simulink model "M10B39_es_V3"  (R2025a)
settings: Solver=ode23tb  StartTime=0.0  StopTime=100  FixedStep=0.001  MaxStep=0.01  RelTol=1e-3  EnableMultiTasking=on
InitFcn:
  | initAll_V3
values from neighbouring files (symbols this model uses):
  acom = 100    [initAll_V1.m]    (also in initAll_V2.m; initAll_V3.m; parameterinit.mat)
  AVm0 = [4.26082678503 4.656135219]    [parameterinit.mat]
  bcom = 50    [initAll_V1.m]    (also in initAll_V2.m; initAll_V3.m; parameterinit.mat)
  commun = 0*commun    [initAll_V1.m]    (also in initAll_V2.m; initAll_V3.m; parameterinit.mat = [0  0  0; 0  0  0; 0  0  0; 0  0  0])
  DataDelay = 0.0*DataDelay    [initAll_V1.m]    (also in initAll_V2.m; initAll_V3.m; parameterinit.mat = [0  0  0; 0  0  0; 0  0  0; 0  0  0])
  ESinit =     [parameterinit.mat]
  fB = 50    [initAll.m]    (also in initAll_V1.m; initAll_V2.m; initAll_V3.m; parameterinit.mat)
  Geninit = Generator_init(opdata,SynMach_in_gidx)    [initAll.m]    (also in initAll_V1.m; initAll_V2.m; initAll_V3.m = Generator_init(opdata_all,SynMach_in_gidx1); parameterinit.mat = )
  lam = 100    [initAll_V1.m]    (also in initAll_V2.m; initAll_V3.m; parameterinit.mat)
  SgridB = 100    [initAll.m]    (also in initAll_V1.m; initAll_V2.m; initAll_V3.m; parameterinit.mat)
  wB = 2*pi*fB    (= 314.159265359)    [initAll.m]    (also in initAll_V1.m; initAll_V2.m; initAll_V3.m; parameterinit.mat)
  Windinit =     [parameterinit.mat]
  YY_load = [3.65450097002 -2.05705688056 0 0 0 0 0 0 0 0 0 0 ... (1521 elements, 39x39)]    [parameterinit.mat]    (also in powerflowcaculate.m = full(YY))
undefined symbols (not defined in the file or in its folder): c1, c2, c3, c4, c5, c6, cp_nom, lambda_nom, P_wind_base, Pelec_base, Pnom
libraries: spsBistableLib x12, simulink_extras x3, slpidlib x2, simulink x1
(part 1 of 7)
settings Model: Creator=m  LastModifiedBy=86182
settings SolverCC: AlgebraicLoopSolver=TrustRegion
settings DataIOCC: LimitDataPoints=on  SaveFormat=Array  SignalLoggingSaveFormat=ModelDataLogs  ReturnWorkspaceOutputs=off  SignalLoggingName=sigsOut
settings OptimizationCC: ExpressionDepthLimit=2147483647.0  LifeSpan=inf
settings DebuggingCC: SaveWithParameterizedLinksMsg=none  UnderspecifiedInitializationDetection=Classic  MergeDetectMultiDrivingBlocksExec=none  SignalResolutionControl=TryResolveAllWithWarning  MultiTaskDSMMsg=warning  MultiTaskCondExecSysMsg=none  FcnCallInpInsideContextMsg=warning  UnconnectedInputMsg=warning  UnconnectedOutputMsg=warning  UnconnectedLineMsg=warning  StateNameClashWarn=warning  SFUnexpectedBacktrackingDiag=warning  SFNoUnconditionalDefaultTransitionDiag=warning  SFExecutionAtInitializationDiag=none  ArithmeticOperatorsInVariantConditions=warning
settings HardwareCC: ProdBitPerPointer=32.0  ProdBitPerSizeT=32.0  ProdBitPerPtrDiffT=32.0  ProdLargestAtomicFloat=None  ProdIntDivRoundTo=Undefined  ProdEndianess=Unspecified  ProdWordSize=32.0  ProdHWDeviceType=32-bit Generic  TargetUnknown=on
settings ModelReferenceCC: EnableRefExpFcnMdlSchedulingChecks=on  PropagateSignalLabelsOutOfModel=off
settings SFSimCC: SimUseLocalCustomCode=off  CustomCodeUndefinedFunction=UseInterfaceOnly
settings RTWCC: RTWUseLocalCustomCode=off  GPUComputeCapability=3.5
settings CodeAppCC: StateflowObjectComments=on
settings GRTTargetCC: TargetLangStandard=C89/C90 (ANSI)  CombineOutputUpdateFcns=off  GRTInterface=on
settings ConfigComp: CovMetricSettings=dw  CovSaveCumulativeToWorkspaceVar=on  CovSaveSingleToWorkspaceVar=on  CovExternalEMLEnable=off  CovSFcnEnable=off

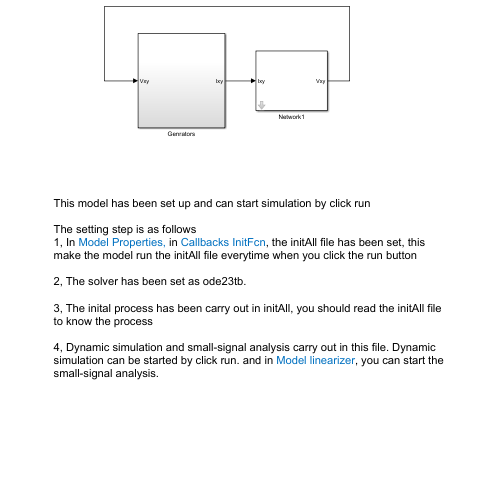
[thumbnail: Simulink's stored preview of the top-level diagram]
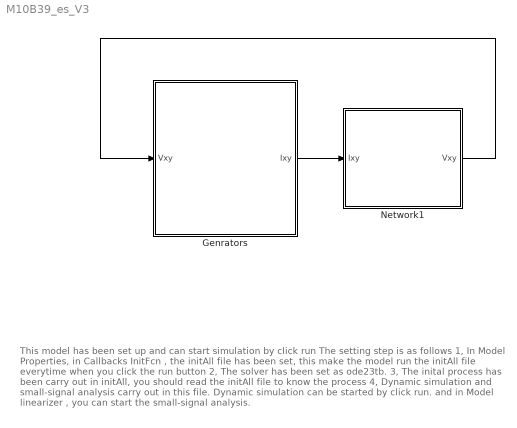
== system M10B39_es_V3 ==
  note: This model has been set up and can start simulation by click run
      |
      | The setting step is as follows
      | 1, In Model Properties, in Callbacks InitFcn , the initAll file has been set, this make the model run the initAll file everytime when you click the run button
      |
      | 2, The solver has been set as ode23tb.
      |
      | 3, The inital process has been carry out in initAll, you should read the initAll file to know the process
      |
      | 4, Dynamic simulation and small-signal analysis carry out in this file. Dynamic simulation can be started by click run. and in Model linearizer , you can start the small-signal analysis.
  Genrators : Subsystem
  Network1 : Subsystem  mask{YY_load=YY_load, ng=12}
  wires:
  Genrators/1(Ixy) -> Network1/1(Ixy)
  Network1/1(Vxy) -> Genrators/1(Vxy)

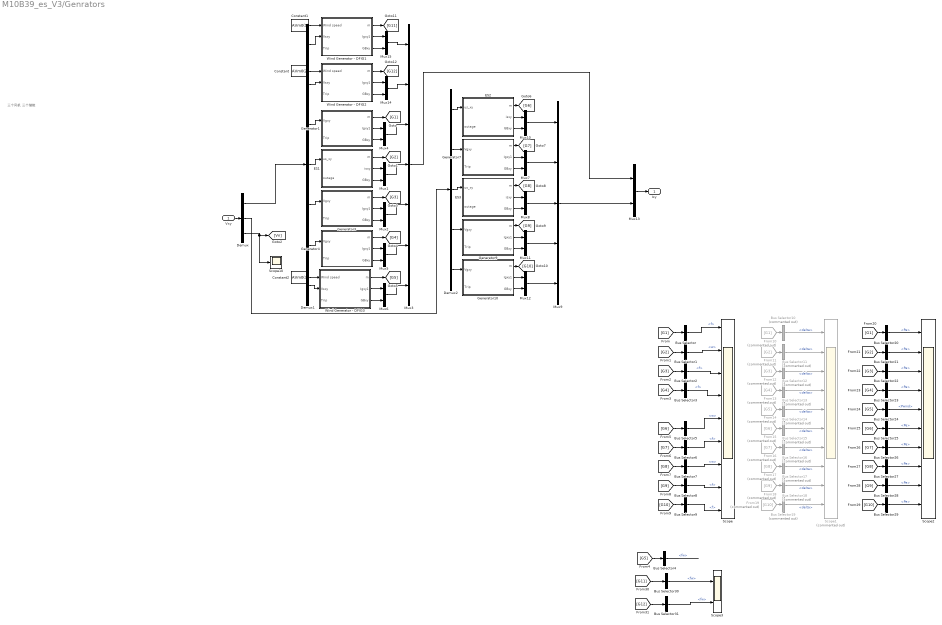
== system M10B39_es_V3/Genrators ==
  note: 三个风机 三个储能
  Vxy : Inport
  Bus Selector{,2..3,6,8..9} (6 alike) : BusSelector  OutputSignals=f
  Bus Selector1 : BusSelector  OutputSignals=w
  Bus Selector{10..19} (10 alike) : BusSelector  Commented=on  OutputSignals=delta
  Bus Selector{20..23,25..29} (9 alike) : BusSelector  OutputSignals=Pe
  Bus Selector24 : BusSelector  OutputSignals=Pwind
  Bus Selector30 : BusSelector  OutputSignals=fw
  Bus Selector31 : BusSelector  OutputSignals=fw
  Bus Selector4 : BusSelector  OutputSignals=fw
  Bus Selector5 : BusSelector  OutputSignals=w
  Bus Selector7 : BusSelector  OutputSignals=w
  Constant : Constant  Value=AVm0(2)
  Constant1 : Constant  Value=AVm0(1)
  Constant2 : Constant  Value=AVm0(3)
  Demux : Demux  Outputs=[14 10 27]
      settings: DisplayOption=none
  Demux1 : Demux  Outputs=7
      settings: DisplayOption=none
  Demux2 : Demux  Outputs=5
      settings: DisplayOption=none
  ES1 : Subsystem  mask{SvscB=ESinit.SvscBi(1), SgridB=SgridB, Kppll_VSC=ESinit.Kppll(1), Kipll_VSC=ESinit.Kipll(1), Dels_hvdc=ESinit.Dels_hvdc(1), Lpr=ESinit.Lpr(1), Rpr=ESinit.Rpr(1), wB=wB, Is_xA_0=ESinit.Isx0(1), Is_yA_0=ESinit.Isy0(1), KpP_VSC_A=ESinit.KpP(1), KiP_VSC_A=ESinit.KiP(1), KpId_VSC_A=ESinit.KpId(1), KiId_VSC_A=ESinit.KiId(1), KpQ_VSC_A=ESinit.KpQ(1), KiQ_VSC_A=ESinit.KiQ(1), KpIq_VSC_A=ESinit.KpIq(1), KiIq_VSC_A=ESinit.KiIq(1), Md_A_0=ESinit.Md0(1), Mq_A_0=ESinit.Mq0(1), Nd_A_0=ESinit.Nd0(1), Nq_A_0=ESinit.Nq0(1), KIR=ESinit.Kir(1), Kdroop=ESinit.Kdroop(1), Kdistributed=ESinit.Kdistributed(1), Kdistributed_d=ESinit.Kdistributed_d(1), Kpac_VSC_A=ESinit.Kpac(1), Kiac_VSC_A=ESinit.Kiac(1), P0=ESinit.P0(1), Q0=ESinit.Q0(1), usd0=ESinit.Usd0(1)}
      mask prompts: Kppll_VSC "Kppll"; Kipll_VSC "Kipll"; KpP_VSC_A "KpP"; KiP_VSC_A "KiP"; KpId_VSC_A "KpId"; KiId_VSC_A "KiId"; KpQ_VSC_A "KpQ"; KiQ_VSC_A "KiQ"; KpIq_VSC_A "KpIq"; KiIq_VSC_A "KiIq"; Kpac_VSC_A "Kpac"; Kiac_VSC_A "Kiac"
      mask DialogControl Container48 Prompt: Base value
      mask DialogControl Container7 Prompt: PLL
      mask DialogControl Container5 Prompt: Control parameter
      mask DialogControl Container8 Prompt: inital value
      mask DialogControl Container9 Prompt: AC side
      mask DialogControl Container10 Prompt: Parameter
      mask DialogControl Container11 Prompt: Initial value
      mask DialogControl Container18 Prompt: Control parameter
      mask DialogControl Container19 Prompt: d_axis_control parameter
      mask DialogControl Container23 Prompt: d_axis_control=1
      mask DialogControl Container26 Prompt: inner current control
      mask DialogControl Container21 Prompt: q_axis_control parameter
      mask DialogControl Container29 Prompt: q_axis_control=1
      mask DialogControl Container31 Prompt: inner current control
      mask DialogControl Container22 Prompt: inital value
      mask DialogControl Container35 Prompt: outer controller
      mask DialogControl Container36 Prompt: inner control
      mask DialogControl Container27 Prompt: Inertia control
      mask DialogControl Container28 Prompt: droop control
      mask DialogControl Container300 Prompt: distributed control
      mask DialogControl Container301 Prompt: Droop distributed control
      mask DialogControl Container40 Prompt: usdq_control
      mask DialogControl Container41 Prompt: PQinitial
      mask DialogControl Container42 Prompt: usd0initial
  ES2 : Subsystem  mask{SvscB=ESinit.SvscBi(2), SgridB=SgridB, Kppll_VSC=ESinit.Kppll(2), Kipll_VSC=ESinit.Kipll(2), Dels_hvdc=ESinit.Dels_hvdc(2), Lpr=ESinit.Lpr(2), Rpr=ESinit.Rpr(2), wB=wB, Is_xA_0=ESinit.Isx0(2), Is_yA_0=ESinit.Isy0(2), KpP_VSC_A=ESinit.KpP(2), KiP_VSC_A=ESinit.KiP(2), KpId_VSC_A=ESinit.KpId(2), KiId_VSC_A=ESinit.KiId(2), KpQ_VSC_A=ESinit.KpQ(2), KiQ_VSC_A=ESinit.KiQ(2), KpIq_VSC_A=ESinit.KpIq(2), KiIq_VSC_A=ESinit.KiIq(2), Md_A_0=ESinit.Md0(2), Mq_A_0=ESinit.Mq0(2), Nd_A_0=ESinit.Nd0(2), Nq_A_0=ESinit.Nq0(2), KIR=ESinit.Kir(2), Kdroop=ESinit.Kdroop(2), Kdistributed=ESinit.Kdistributed(2), Kdistributed_d=ESinit.Kdistributed_d(2), Kpac_VSC_A=ESinit.Kpac(2), Kiac_VSC_A=ESinit.Kiac(2), P0=ESinit.P0(2), Q0=ESinit.Q0(2), usd0=ESinit.Usd0(2)}
      mask prompts: Kppll_VSC "Kppll"; Kipll_VSC "Kipll"; KpP_VSC_A "KpP"; KiP_VSC_A "KiP"; KpId_VSC_A "KpId"; KiId_VSC_A "KiId"; KpQ_VSC_A "KpQ"; KiQ_VSC_A "KiQ"; KpIq_VSC_A "KpIq"; KiIq_VSC_A "KiIq"; Kpac_VSC_A "Kpac"; Kiac_VSC_A "Kiac"
      mask DialogControl Container48 Prompt: Base value
      mask DialogControl Container7 Prompt: PLL
      mask DialogControl Container5 Prompt: Control parameter
      mask DialogControl Container8 Prompt: inital value
      mask DialogControl Container9 Prompt: AC side
      mask DialogControl Container10 Prompt: Parameter
      mask DialogControl Container11 Prompt: Initial value
      mask DialogControl Container18 Prompt: Control parameter
      mask DialogControl Container19 Prompt: d_axis_control parameter
      mask DialogControl Container23 Prompt: d_axis_control=1
      mask DialogControl Container26 Prompt: inner current control
      mask DialogControl Container21 Prompt: q_axis_control parameter
      mask DialogControl Container29 Prompt: q_axis_control=1
      mask DialogControl Container31 Prompt: inner current control
      mask DialogControl Container22 Prompt: inital value
      mask DialogControl Container35 Prompt: outer controller
      mask DialogControl Container36 Prompt: inner control
      mask DialogControl Container27 Prompt: Inertia control
      mask DialogControl Container28 Prompt: droop control
      mask DialogControl Container300 Prompt: distributed control
      mask DialogControl Container301 Prompt: Droop distributed control
      mask DialogControl Container40 Prompt: usdq_control
      mask DialogControl Container41 Prompt: PQinitial
      mask DialogControl Container42 Prompt: usd0initial
  ES3 : Subsystem  mask{SvscB=ESinit.SvscBi(3), SgridB=SgridB, Kppll_VSC=ESinit.Kppll(3), Kipll_VSC=ESinit.Kipll(3), Dels_hvdc=ESinit.Dels_hvdc(3), Lpr=ESinit.Lpr(3), Rpr=ESinit.Rpr(3), wB=wB, Is_xA_0=ESinit.Isx0(3), Is_yA_0=ESinit.Isy0(3), KpP_VSC_A=ESinit.KpP(3), KiP_VSC_A=ESinit.KiP(3), KpId_VSC_A=ESinit.KpId(3), KiId_VSC_A=ESinit.KiId(3), KpQ_VSC_A=ESinit.KpQ(3), KiQ_VSC_A=ESinit.KiQ(3), KpIq_VSC_A=ESinit.KpIq(3), KiIq_VSC_A=ESinit.KiIq(3), Md_A_0=ESinit.Md0(3), Mq_A_0=ESinit.Mq0(3), Nd_A_0=ESinit.Nd0(3), Nq_A_0=ESinit.Nq0(3), KIR=ESinit.Kir(3), Kdroop=ESinit.Kdroop(3), Kdistributed=ESinit.Kdistributed(3), Kdistributed_d=ESinit.Kdistributed_d(3), Kpac_VSC_A=ESinit.Kpac(3), Kiac_VSC_A=ESinit.Kiac(3), P0=ESinit.P0(3), Q0=ESinit.Q0(3), usd0=ESinit.Usd0(3)}
      mask prompts: Kppll_VSC "Kppll"; Kipll_VSC "Kipll"; KpP_VSC_A "KpP"; KiP_VSC_A "KiP"; KpId_VSC_A "KpId"; KiId_VSC_A "KiId"; KpQ_VSC_A "KpQ"; KiQ_VSC_A "KiQ"; KpIq_VSC_A "KpIq"; KiIq_VSC_A "KiIq"; Kpac_VSC_A "Kpac"; Kiac_VSC_A "Kiac"
      mask DialogControl Container48 Prompt: Base value
      mask DialogControl Container7 Prompt: PLL
      mask DialogControl Container5 Prompt: Control parameter
      mask DialogControl Container8 Prompt: inital value
      mask DialogControl Container9 Prompt: AC side
      mask DialogControl Container10 Prompt: Parameter
      mask DialogControl Container11 Prompt: Initial value
      mask DialogControl Container18 Prompt: Control parameter
      mask DialogControl Container19 Prompt: d_axis_control parameter
      mask DialogControl Container23 Prompt: d_axis_control=1
      mask DialogControl Container26 Prompt: inner current control
      mask DialogControl Container21 Prompt: q_axis_control parameter
      mask DialogControl Container29 Prompt: q_axis_control=1
      mask DialogControl Container31 Prompt: inner current control
      mask DialogControl Container22 Prompt: inital value
      mask DialogControl Container35 Prompt: outer controller
      mask DialogControl Container36 Prompt: inner control
      mask DialogControl Container27 Prompt: Inertia control
      mask DialogControl Container28 Prompt: droop control
      mask DialogControl Container300 Prompt: distributed control
      mask DialogControl Container301 Prompt: Droop distributed control
      mask DialogControl Container40 Prompt: usdq_control
      mask DialogControl Container41 Prompt: PQinitial
      mask DialogControl Container42 Prompt: usd0initial
  From10 : From  Commented=on  GotoTag=G1
  From11 : From  Commented=on  GotoTag=G2
  From12 : From  Commented=on  GotoTag=G3
  From13 : From  Commented=on  GotoTag=G4
  From14 : From  Commented=on  GotoTag=G5
  From15 : From  Commented=on  GotoTag=G6
  From16 : From  Commented=on  GotoTag=G7
  From17 : From  Commented=on  GotoTag=G8
  From18 : From  Commented=on  GotoTag=G9
  From19 : From  Commented=on  GotoTag=G10
  Generator1 : Subsystem  mask{wB=wB, SgenB=Geninit.SgenB(1), SgridB=SgridB, Xq=Geninit.Xq(1), Xq1=Geninit.Xq1(1), Xq11=Geninit.Xq11(1), Tq0=Geninit.Tq0(1), Tq10=Geninit.Tq10(1), Eq10=Geninit.Eq1(1), Eq110=Geninit.Eq11(1), Xd=Geninit.Xd(1), Xd1=Geninit.Xd1(1), Xd11=Geninit.Xd11(1), Td0=Geninit.Td0(1), Td10=Geninit.Td10(1), Ed10=Geninit.Ed1(1), Ed110=Geninit.Ed11(1), H=Geninit.Tj(1), D=Geninit.D(1), delta0=Geninit.Delta(1), w0=1, Pm0=Geninit.Pm0(1), Ka=Geninit.Ka(1), Tb=Geninit.Tb(1), Tc=Geninit.Tc(1), Efmax=Geninit.Efmax(1), Efmin=Geninit.Efmin(1), Vref=Geninit.Vref(1), Ef10=Geninit.Vf1(1), S_PSS=Geninit.EnablePSS(1), Kpss=Geninit.kpss(1), Tw_P=Geninit.Tw_P(1), T1_P=Geninit.T1_P(1), T2_P=Geninit.T2_P(1), T3_P=Geninit.T3_P(1), T4_P=Geninit.T4_P(1), Upmax=Geninit.Upmax(1), Upmin=Geninit.Upmin(1), S_Gov=Geninit.Enablegov(1), a_G=Geninit.a_G(1), b_G=Geninit.b_G(1), Tg_G=Geninit.Tg_G(1), dPmax=Geninit.dPmax(1), dPmin=Geninit.dPmin(1)}
      mask prompts: S_PSS "Enable PSS"; Tw_P "Tw"; T1_P "T1"; T2_P "T2"; T3_P "T3"; T4_P "T4"; S_Gov "Enable Governor"; a_G "a"; b_G "b"; Tg_G "Tg"
      mask help: This is a six-order synchronous generator with exciter system, governor and PSS.
      mask DialogControl Container6 Prompt: Machine parameter
      mask DialogControl Container3 Prompt: q axis parameter
      mask DialogControl ParameterGroupVar Prompt: d axis parameter
      mask DialogControl Container4 Prompt: machine parameter
      mask DialogControl Container12 Prompt: Excitation System parameter
      mask DialogControl Container20 Prompt: parameter
      mask DialogControl Container21 Prompt: inital value
      mask DialogControl Container10 Prompt: PSS parameter
      mask DialogControl Container13 Prompt: Governor parameter
  Generator10 : Subsystem  mask{wB=wB, SgenB=Geninit.SgenB(10), SgridB=SgridB, Xq=Geninit.Xq(10), Xq1=Geninit.Xq1(10), Xq11=Geninit.Xq11(10), Tq0=Geninit.Tq0(10), Tq10=Geninit.Tq10(10), Eq10=Geninit.Eq1(10), Eq110=Geninit.Eq11(10), Xd=Geninit.Xd(10), Xd1=Geninit.Xd1(10), Xd11=Geninit.Xd11(10), Td0=Geninit.Td0(10), Td10=Geninit.Td10(10), Ed10=Geninit.Ed1(10), Ed110=Geninit.Ed11(10), H=Geninit.Tj(10), D=Geninit.D(10), delta0=Geninit.Delta(10), w0=1, Pm0=Geninit.Pm0(10), Ka=Geninit.Ka(10), Tb=Geninit.Tb(10), Tc=Geninit.Tc(10), Efmax=Geninit.Efmax(10), Efmin=Geninit.Efmin(10), Vref=Geninit.Vref(10), Ef10=Geninit.Vf1(10), S_PSS=Geninit.EnablePSS(10), Kpss=Geninit.kpss(10), Tw_P=Geninit.Tw_P(10), T1_P=Geninit.T1_P(10), T2_P=Geninit.T2_P(10), T3_P=Geninit.T3_P(10), T4_P=Geninit.T4_P(10), Upmax=Geninit.Upmax(10), Upmin=Geninit.Upmin(10), S_Gov=Geninit.Enablegov(10), a_G=Geninit.a_G(10), b_G=Geninit.b_G(10), Tg_G=Geninit.Tg_G(10), dPmax=Geninit.dPmax(10), dPmin=Geninit.dPmin(10)}
      mask prompts: S_PSS "Enable PSS"; Tw_P "Tw"; T1_P "T1"; T2_P "T2"; T3_P "T3"; T4_P "T4"; S_Gov "Enable Governor"; a_G "a"; b_G "b"; Tg_G "Tg"
      mask help: This is a six-order synchronous generator with exciter system, governor and PSS.
      mask DialogControl Container6 Prompt: Machine parameter
      mask DialogControl Container3 Prompt: q axis parameter
      mask DialogControl ParameterGroupVar Prompt: d axis parameter
      mask DialogControl Container4 Prompt: machine parameter
      mask DialogControl Container12 Prompt: Excitation System parameter
      mask DialogControl Container20 Prompt: parameter
      mask DialogControl Container21 Prompt: inital value
      mask DialogControl Container10 Prompt: PSS parameter
      mask DialogControl Container13 Prompt: Governor parameter
  Generator3 : Subsystem  mask{wB=wB, SgenB=Geninit.SgenB(3), SgridB=SgridB, Xq=Geninit.Xq(3), Xq1=Geninit.Xq1(3), Xq11=Geninit.Xq11(3), Tq0=Geninit.Tq0(3), Tq10=Geninit.Tq10(3), Eq10=Geninit.Eq1(3), Eq110=Geninit.Eq11(3), Xd=Geninit.Xd(3), Xd1=Geninit.Xd1(3), Xd11=Geninit.Xd11(3), Td0=Geninit.Td0(3), Td10=Geninit.Td10(3), Ed10=Geninit.Ed1(3), Ed110=Geninit.Ed11(3), H=Geninit.Tj(3), D=Geninit.D(3), delta0=Geninit.Delta(3), w0=1, Pm0=Geninit.Pm0(3), Ka=Geninit.Ka(3), Tb=Geninit.Tb(3), Tc=Geninit.Tc(3), Efmax=Geninit.Efmax(3), Efmin=Geninit.Efmin(3), Vref=Geninit.Vref(3), Ef10=Geninit.Vf1(3), S_PSS=Geninit.EnablePSS(3), Kpss=Geninit.kpss(3), Tw_P=Geninit.Tw_P(3), T1_P=Geninit.T1_P(3), T2_P=Geninit.T2_P(3), T3_P=Geninit.T3_P(3), T4_P=Geninit.T4_P(3), Upmax=Geninit.Upmax(3), Upmin=Geninit.Upmin(3), S_Gov=Geninit.Enablegov(3), a_G=Geninit.a_G(3), b_G=Geninit.b_G(3), Tg_G=Geninit.Tg_G(3), dPmax=Geninit.dPmax(3), dPmin=Geninit.dPmin(3)}
      mask prompts: S_PSS "Enable PSS"; Tw_P "Tw"; T1_P "T1"; T2_P "T2"; T3_P "T3"; T4_P "T4"; S_Gov "Enable Governor"; a_G "a"; b_G "b"; Tg_G "Tg"
      mask help: This is a six-order synchronous generator with exciter system, governor and PSS.
      mask DialogControl Container6 Prompt: Machine parameter
      mask DialogControl Container3 Prompt: q axis parameter
      mask DialogControl ParameterGroupVar Prompt: d axis parameter
      mask DialogControl Container4 Prompt: machine parameter
      mask DialogControl Container12 Prompt: Excitation System parameter
      mask DialogControl Container20 Prompt: parameter
      mask DialogControl Container21 Prompt: inital value
      mask DialogControl Container10 Prompt: PSS parameter
      mask DialogControl Container13 Prompt: Governor parameter
  Generator4 : Subsystem  mask{wB=wB, SgenB=Geninit.SgenB(4), SgridB=SgridB, Xq=Geninit.Xq(4), Xq1=Geninit.Xq1(4), Xq11=Geninit.Xq11(4), Tq0=Geninit.Tq0(4), Tq10=Geninit.Tq10(4), Eq10=Geninit.Eq1(4), Eq110=Geninit.Eq11(4), Xd=Geninit.Xd(4), Xd1=Geninit.Xd1(4), Xd11=Geninit.Xd11(4), Td0=Geninit.Td0(4), Td10=Geninit.Td10(4), Ed10=Geninit.Ed1(4), Ed110=Geninit.Ed11(4), H=Geninit.Tj(4), D=Geninit.D(4), delta0=Geninit.Delta(4), w0=1, Pm0=Geninit.Pm0(4), Ka=Geninit.Ka(4), Tb=Geninit.Tb(4), Tc=Geninit.Tc(4), Efmax=Geninit.Efmax(4), Efmin=Geninit.Efmin(4), Vref=Geninit.Vref(4), Ef10=Geninit.Vf1(4), S_PSS=Geninit.EnablePSS(4), Kpss=Geninit.kpss(4), Tw_P=Geninit.Tw_P(4), T1_P=Geninit.T1_P(4), T2_P=Geninit.T2_P(4), T3_P=Geninit.T3_P(4), T4_P=Geninit.T4_P(4), Upmax=Geninit.Upmax(4), Upmin=Geninit.Upmin(4), S_Gov=Geninit.Enablegov(4), a_G=Geninit.a_G(4), b_G=Geninit.b_G(4), Tg_G=Geninit.Tg_G(4), dPmax=Geninit.dPmax(4), dPmin=Geninit.dPmin(4)}
      mask prompts: S_PSS "Enable PSS"; Tw_P "Tw"; T1_P "T1"; T2_P "T2"; T3_P "T3"; T4_P "T4"; S_Gov "Enable Governor"; a_G "a"; b_G "b"; Tg_G "Tg"
      mask help: This is a six-order synchronous generator with exciter system, governor and PSS.
      mask DialogControl Container6 Prompt: Machine parameter
      mask DialogControl Container3 Prompt: q axis parameter
      mask DialogControl ParameterGroupVar Prompt: d axis parameter
      mask DialogControl Container4 Prompt: machine parameter
      mask DialogControl Container12 Prompt: Excitation System parameter
      mask DialogControl Container20 Prompt: parameter
      mask DialogControl Container21 Prompt: inital value
      mask DialogControl Container10 Prompt: PSS parameter
      mask DialogControl Container13 Prompt: Governor parameter
  Generator7 : Subsystem  mask{wB=wB, SgenB=Geninit.SgenB(7), SgridB=SgridB, Xq=Geninit.Xq(7), Xq1=Geninit.Xq1(7), Xq11=Geninit.Xq11(7), Tq0=Geninit.Tq0(7), Tq10=Geninit.Tq10(7), Eq10=Geninit.Eq1(7), Eq110=Geninit.Eq11(7), Xd=Geninit.Xd(7), Xd1=Geninit.Xd1(7), Xd11=Geninit.Xd11(7), Td0=Geninit.Td0(7), Td10=Geninit.Td10(7), Ed10=Geninit.Ed1(7), Ed110=Geninit.Ed11(7), H=Geninit.Tj(7), D=Geninit.D(7), delta0=Geninit.Delta(7), w0=1, Pm0=Geninit.Pm0(7), Ka=Geninit.Ka(7), Tb=Geninit.Tb(7), Tc=Geninit.Tc(7), Efmax=Geninit.Efmax(7), Efmin=Geninit.Efmin(7), Vref=Geninit.Vref(7), Ef10=Geninit.Vf1(7), S_PSS=Geninit.EnablePSS(7), Kpss=Geninit.kpss(7), Tw_P=Geninit.Tw_P(7), T1_P=Geninit.T1_P(7), T2_P=Geninit.T2_P(7), T3_P=Geninit.T3_P(7), T4_P=Geninit.T4_P(7), Upmax=Geninit.Upmax(7), Upmin=Geninit.Upmin(7), S_Gov=Geninit.Enablegov(7), a_G=Geninit.a_G(7), b_G=Geninit.b_G(7), Tg_G=Geninit.Tg_G(7), dPmax=Geninit.dPmax(7), dPmin=Geninit.dPmin(7)}
      mask prompts: S_PSS "Enable PSS"; Tw_P "Tw"; T1_P "T1"; T2_P "T2"; T3_P "T3"; T4_P "T4"; S_Gov "Enable Governor"; a_G "a"; b_G "b"; Tg_G "Tg"
      mask help: This is a six-order synchronous generator with exciter system, governor and PSS.
      mask DialogControl Container6 Prompt: Machine parameter
      mask DialogControl Container3 Prompt: q axis parameter
      mask DialogControl ParameterGroupVar Prompt: d axis parameter
      mask DialogControl Container4 Prompt: machine parameter
      mask DialogControl Container12 Prompt: Excitation System parameter
      mask DialogControl Container20 Prompt: parameter
      mask DialogControl Container21 Prompt: inital value
      mask DialogControl Container10 Prompt: PSS parameter
      mask DialogControl Container13 Prompt: Governor parameter
  Generator9 : Subsystem  mask{wB=wB, SgenB=Geninit.SgenB(9), SgridB=SgridB, Xq=Geninit.Xq(9), Xq1=Geninit.Xq1(9), Xq11=Geninit.Xq11(9), Tq0=Geninit.Tq0(9), Tq10=Geninit.Tq10(9), Eq10=Geninit.Eq1(9), Eq110=Geninit.Eq11(9), Xd=Geninit.Xd(9), Xd1=Geninit.Xd1(9), Xd11=Geninit.Xd11(9), Td0=Geninit.Td0(9), Td10=Geninit.Td10(9), Ed10=Geninit.Ed1(9), Ed110=Geninit.Ed11(9), H=Geninit.Tj(9), D=Geninit.D(9), delta0=Geninit.Delta(9), w0=1, Pm0=Geninit.Pm0(9), Ka=Geninit.Ka(9), Tb=Geninit.Tb(9), Tc=Geninit.Tc(9), Efmax=Geninit.Efmax(9), Efmin=Geninit.Efmin(9), Vref=Geninit.Vref(9), Ef10=Geninit.Vf1(9), S_PSS=Geninit.EnablePSS(9), Kpss=Geninit.kpss(9), Tw_P=Geninit.Tw_P(9), T1_P=Geninit.T1_P(9), T2_P=Geninit.T2_P(9), T3_P=Geninit.T3_P(9), T4_P=Geninit.T4_P(9), Upmax=Geninit.Upmax(9), Upmin=Geninit.Upmin(9), S_Gov=Geninit.Enablegov(9), a_G=Geninit.a_G(9), b_G=Geninit.b_G(9), Tg_G=Geninit.Tg_G(9), dPmax=Geninit.dPmax(9), dPmin=Geninit.dPmin(9)}
      mask prompts: S_PSS "Enable PSS"; Tw_P "Tw"; T1_P "T1"; T2_P "T2"; T3_P "T3"; T4_P "T4"; S_Gov "Enable Governor"; a_G "a"; b_G "b"; Tg_G "Tg"
      mask help: This is a six-order synchronous generator with exciter system, governor and PSS.
      mask DialogControl Container6 Prompt: Machine parameter
      mask DialogControl Container3 Prompt: q axis parameter
      mask DialogControl ParameterGroupVar Prompt: d axis parameter
      mask DialogControl Container4 Prompt: machine parameter
      mask DialogControl Container12 Prompt: Excitation System parameter
      mask DialogControl Container20 Prompt: parameter
      mask DialogControl Container21 Prompt: inital value
      mask DialogControl Container10 Prompt: PSS parameter
      mask DialogControl Container13 Prompt: Governor parameter
  Mux{1..2,4..8,10..15} (13 alike) : Mux  Inputs=2
  Mux3 : Mux  Inputs=7
  Mux9 : Mux  Inputs=5
  Scope : Scope  NumInputPorts=9
      settings: ActiveDisplayYMinimum=-1.6197293838194131  ActiveDisplayYMaximum=1.2914865659117496
  Scope1 : Scope  Commented=on  NumInputPorts=10
      settings: ActiveDisplayYMinimum=-0.16939  ActiveDisplayYMaximum=1.28958  DataLoggingVariableName=ScopeData2
  Scope10 : Scope
      settings: ActiveDisplayYMinimum=0.98473  ActiveDisplayYMaximum=1.07242  DataLoggingVariableName=ScopeData4
  Scope2 : Scope  NumInputPorts=10
      settings: ActiveDisplayYMinimum=1.2239  ActiveDisplayYMaximum=10.49404  DataLoggingVariableName=ScopeData3
  Scope3 : Scope  NumInputPorts=2
      settings: ActiveDisplayYMinimum=-0.81770922581962058  ActiveDisplayYMaximum=1.2019676917577355
  Wind Generator - DFIG1 : Subsystem  mask{NN=Windinit.NN(1), SwgBi=Windinit.SwgBi(1), SmecBi=100, SgridB=SgridB, Atheta=Windinit.Atheta(1), Kppll=Windinit.Kppll_wind(1), Kipll=Windinit.Kipll_wind(1), pitch=[500 45 2], Srotors=1.3, H=Windinit.H(1), Wr0=Windinit.Wr0(1), Xa=Windinit.Xa(1), Xa1=Windinit.Xa1(1), Lm=Windinit.Lm(1), Lr=Windinit.Lr(1), Rs=Windinit.Rs(1), Ls=Windinit.Ls(1), Ta0=Windinit.Ta0(1), NPf=Windinit.NPf(1), Za=Windinit.Za{1}, Ex0=Windinit.Ex_ref(1), Ey0=Windinit.Ey_ref(1), wB=wB, KpP_rw=Windinit.KpP_rw(1), KiP_rw=Windinit.KiP_rw(1), KpId_rw=Windinit.KpId_rw(1), KiId_rw=Windinit.KiId_rw(1), KpQ_rw=Windinit.KpQ_rw(1), KiQ_rw=Windinit.KiQ_rw(1), KpIq_rw=Windinit.KpIq_rw(1), KiIq_rw=Windinit.KiIq_rw(1), Ird_ref=Windinit.Ird_ref(1), Irq_ref=Windinit.Irq_ref(1), Qs0=Windinit.Qs0(1), KpDC_gw=Windinit.KpDC_gw(1), KiDC_gw=Windinit.KiDC_gw(1), KpId_gw=Windinit.KpId_gw(1), KiId_gw=Windinit.KiId_gw(1), KpIq_gw=Windinit.KpIq_gw(1), KiIq_gw=Windinit.KiIq_gw(1), Vdc_w=Windinit.Vdc_w(1), Icd_ref=Windinit.Icd_ref(1), Icq_ref=Windinit.Icq_ref(1), Vcd_ref=Windinit.Vcd_ref(1), Vcq_ref=Windinit.Vcq_ref(1), Lg=Windinit.Lg(1), Rg=Windinit.Rg(1), Icx0=Windinit.Icx0(1), Icy0=Windinit.Icy0(1), C_w=Windinit.C_w(1), Vdc0=Windinit.Vdc0(1)}
      mask prompts: pitch "pitch_gain，pitch_max，pitch_rate"; Srotors "Start Rotor Speed"; Ex0 "Ex"; Ey0 "Ey"
      mask init:
      | pitch_gain=pitch(1);
      | pitch_max=pitch(2);
      | pitch_rate=pitch(3);
      | 
      | %该风机模型的基准容量
      | 
      | SwgeqB=SwgBi.*NN;
      mask DialogControl Container4 Prompt: PLL/Wind turbine
      mask DialogControl Container31 Prompt: Base value
      mask DialogControl Container23 Prompt: PLL
      mask DialogControl Container6 Prompt: inital value
      mask DialogControl Container5 Prompt: PI parameter
      mask DialogControl Container24 Prompt: Wind turbine
      mask DialogControl Container25 Prompt: pitch control
      mask DialogControl Container7 Prompt: Machine parameter
      mask DialogControl Container8 Prompt: Rotor
      mask DialogControl Container9 Prompt: Machine
      mask DialogControl Container10 Prompt: parameter
      mask DialogControl Container11 Prompt: inital value
      mask DialogControl Container12 Prompt: Rotor side control
      mask DialogControl Container13 Prompt: Control parameter
      mask DialogControl Container14 Prompt: Initial value
      mask DialogControl Container15 Prompt: reactive power
      mask DialogControl Container16 Prompt: Grid side control
      mask DialogControl Container17 Prompt: parameter
      mask DialogControl Container18 Prompt: reference
      mask DialogControl Container19 Prompt: inital value
      mask DialogControl Container20 Prompt: converter function
      mask DialogControl Container21 Prompt: inital value
      mask DialogControl Container22 Prompt: DC function
  Wind Generator - DFIG2 : Subsystem  mask{NN=Windinit.NN(2), SwgBi=Windinit.SwgBi(2), SmecBi=100, SgridB=SgridB, Atheta=Windinit.Atheta(2), Kppll=Windinit.Kppll_wind(2), Kipll=Windinit.Kipll_wind(2), pitch=[500 45 2], Srotors=1.3, H=Windinit.H(2), Wr0=Windinit.Wr0(2), Xa=Windinit.Xa(2), Xa1=Windinit.Xa1(2), Lm=Windinit.Lm(2), Lr=Windinit.Lr(2), Rs=Windinit.Rs(2), Ls=Windinit.Ls(2), Ta0=Windinit.Ta0(2), NPf=Windinit.NPf(2), Za=Windinit.Za{2}, Ex0=Windinit.Ex_ref(2), Ey0=Windinit.Ey_ref(2), wB=wB, KpP_rw=Windinit.KpP_rw(2), KiP_rw=Windinit.KiP_rw(2), KpId_rw=Windinit.KpId_rw(2), KiId_rw=Windinit.KiId_rw(2), KpQ_rw=Windinit.KpQ_rw(2), KiQ_rw=Windinit.KiQ_rw(2), KpIq_rw=Windinit.KpIq_rw(2), KiIq_rw=Windinit.KiIq_rw(2), Ird_ref=Windinit.Ird_ref(2), Irq_ref=Windinit.Irq_ref(2), Qs0=Windinit.Qs0(2), KpDC_gw=Windinit.KpDC_gw(2), KiDC_gw=Windinit.KiDC_gw(2), KpId_gw=Windinit.KpId_gw(2), KiId_gw=Windinit.KiId_gw(2), KpIq_gw=Windinit.KpIq_gw(2), KiIq_gw=Windinit.KiIq_gw(2), Vdc_w=Windinit.Vdc_w(2), Icd_ref=Windinit.Icd_ref(2), Icq_ref=Windinit.Icq_ref(2), Vcd_ref=Windinit.Vcd_ref(2), Vcq_ref=Windinit.Vcq_ref(2), Lg=Windinit.Lg(2), Rg=Windinit.Rg(2), Icx0=Windinit.Icx0(2), Icy0=Windinit.Icy0(2), C_w=Windinit.C_w(2), Vdc0=Windinit.Vdc0(2)}
      mask prompts: pitch "pitch_gain，pitch_max，pitch_rate"; Srotors "Start Rotor Speed"; Ex0 "Ex"; Ey0 "Ey"
      mask init:
      | pitch_gain=pitch(1);
      | pitch_max=pitch(2);
      | pitch_rate=pitch(3);
      | 
      | %该风机模型的基准容量
      | 
      | SwgeqB=SwgBi.*NN;
      mask DialogControl Container4 Prompt: PLL/Wind turbine
      mask DialogControl Container31 Prompt: Base value
      mask DialogControl Container23 Prompt: PLL
      mask DialogControl Container6 Prompt: inital value
      mask DialogControl Container5 Prompt: PI parameter
      mask DialogControl Container24 Prompt: Wind turbine
      mask DialogControl Container25 Prompt: pitch control
      mask DialogControl Container7 Prompt: Machine parameter
      mask DialogControl Container8 Prompt: Rotor
      mask DialogControl Container9 Prompt: Machine
      mask DialogControl Container10 Prompt: parameter
      mask DialogControl Container11 Prompt: inital value
      mask DialogControl Container12 Prompt: Rotor side control
      mask DialogControl Container13 Prompt: Control parameter
      mask DialogControl Container14 Prompt: Initial value
      mask DialogControl Container15 Prompt: reactive power
      mask DialogControl Container16 Prompt: Grid side control
      mask DialogControl Container17 Prompt: parameter
      mask DialogControl Container18 Prompt: reference
      mask DialogControl Container19 Prompt: inital value
      mask DialogControl Container20 Prompt: converter function
      mask DialogControl Container21 Prompt: inital value
      mask DialogControl Container22 Prompt: DC function
  Wind Generator - DFIG3 : Subsystem  mask{NN=Windinit.NN(3), SwgBi=Windinit.SwgBi(3), SmecBi=100, SgridB=SgridB, Atheta=Windinit.Atheta(3), Kppll=Windinit.Kppll_wind(3), Kipll=Windinit.Kipll_wind(3), pitch=[500 45 2], Srotors=1.3, H=Windinit.H(3), Wr0=Windinit.Wr0(3), Xa=Windinit.Xa(3), Xa1=Windinit.Xa1(3), Lm=Windinit.Lm(3), Lr=Windinit.Lr(3), Rs=Windinit.Rs(3), Ls=Windinit.Ls(3), Ta0=Windinit.Ta0(3), NPf=Windinit.NPf(3), Za=Windinit.Za{3}, Ex0=Windinit.Ex_ref(3), Ey0=Windinit.Ey_ref(3), wB=wB, KpP_rw=Windinit.KpP_rw(3), KiP_rw=Windinit.KiP_rw(3), KpId_rw=Windinit.KpId_rw(3), KiId_rw=Windinit.KiId_rw(3), KpQ_rw=Windinit.KpQ_rw(3), KiQ_rw=Windinit.KiQ_rw(3), KpIq_rw=Windinit.KpIq_rw(3), KiIq_rw=Windinit.KiIq_rw(3), Ird_ref=Windinit.Ird_ref(3), Irq_ref=Windinit.Irq_ref(3), Qs0=Windinit.Qs0(3), KpDC_gw=Windinit.KpDC_gw(3), KiDC_gw=Windinit.KiDC_gw(3), KpId_gw=Windinit.KpId_gw(3), KiId_gw=Windinit.KiId_gw(3), KpIq_gw=Windinit.KpIq_gw(3), KiIq_gw=Windinit.KiIq_gw(3), Vdc_w=Windinit.Vdc_w(3), Icd_ref=Windinit.Icd_ref(3), Icq_ref=Windinit.Icq_ref(3), Vcd_ref=Windinit.Vcd_ref(3), Vcq_ref=Windinit.Vcq_ref(3), Lg=Windinit.Lg(3), Rg=Windinit.Rg(3), Icx0=Windinit.Icx0(3), Icy0=Windinit.Icy0(3), C_w=Windinit.C_w(3), Vdc0=Windinit.Vdc0(3)}
      mask prompts: pitch "pitch_gain，pitch_max，pitch_rate"; Srotors "Start Rotor Speed"; Ex0 "Ex"; Ey0 "Ey"
      mask init:
      | pitch_gain=pitch(1);
      | pitch_max=pitch(2);
      | pitch_rate=pitch(3);
      | 
      | %该风机模型的基准容量
      | 
      | SwgeqB=SwgBi.*NN;
      mask DialogControl Container4 Prompt: PLL/Wind turbine
      mask DialogControl Container31 Prompt: Base value
      mask DialogControl Container23 Prompt: PLL
      mask DialogControl Container6 Prompt: inital value
      mask DialogControl Container5 Prompt: PI parameter
      mask DialogControl Container24 Prompt: Wind turbine
      mask DialogControl Container25 Prompt: pitch control
      mask DialogControl Container7 Prompt: Machine parameter
      mask DialogControl Container8 Prompt: Rotor
      mask DialogControl Container9 Prompt: Machine
      mask DialogControl Container10 Prompt: parameter
      mask DialogControl Container11 Prompt: inital value
      mask DialogControl Container12 Prompt: Rotor side control
      mask DialogControl Container13 Prompt: Control parameter
      mask DialogControl Container14 Prompt: Initial value
      mask DialogControl Container15 Prompt: reactive power
      mask DialogControl Container16 Prompt: Grid side control
      mask DialogControl Container17 Prompt: parameter
      mask DialogControl Container18 Prompt: reference
      mask DialogControl Container19 Prompt: inital value
      mask DialogControl Container20 Prompt: converter function
      mask DialogControl Container21 Prompt: inital value
      mask DialogControl Container22 Prompt: DC function
  Ixy : Outport
  wires:
  Generator1/2(Igxy1) -> Mux4/1
  Generator1/3(GBxy) -> Mux4/2
  Generator3/2(Igxy1) -> Mux2/1
  Generator3/3(GBxy) -> Mux2/2
  Generator4/3(GBxy) -> Mux5/2
  Wind Generator - DFIG3/2(Igxy1) -> Mux6/1
  Wind Generator - DFIG3/3(GBxy) -> Mux6/2
  ES2/2(isxy) -> Mux10/1
  ES2/3(GBxy) -> Mux10/2
  Generator7/2(Igxy1) -> Mux7/1
  Generator7/3(GBxy) -> Mux7/2
  ES3/2(isxy) -> Mux8/1
  ES3/3(GBxy) -> Mux8/2
  Generator9/2(Igxy1) -> Mux11/1
  Generator9/3(GBxy) -> Mux11/2
  Generator10/2(Igxy1) -> Mux12/1
  Generator10/3(GBxy) -> Mux12/2
  Mux10/1 -> Mux9/1
  Mux7/1 -> Mux9/2
  Mux8/1 -> Mux9/3
  Mux11/1 -> Mux9/4
  Mux12/1 -> Mux9/5
  Demux2/2 -> Generator7/1(Vgxy)
  Demux2/4 -> Generator9/1(Vgxy)
  Demux2/5 -> Generator10/1(Vgxy)
  Mux13/1 -> Ixy/1
  Mux9/1 -> Mux13/2
  Mux3/1 -> Mux13/1
  Vxy/1 -> Demux/1
  Demux/1 -> Demux1/1
  Demux/2 -> Demux2/1
  Demux/3 -> [Vn], Scope10/1
  ES1/2(isxy) -> Mux1/1
  ES1/3(GBxy) -> Mux1/2
  Generator4/2(Igxy1) -> Mux5/1
  Generator1/1(m) -> [G1]
  ES1/1(m) -> [G2]
  Generator3/1(m) -> [G3]
  Generator4/1(m) -> [G4]
  Wind Generator - DFIG3/1(m) -> [G5]
  ES2/1(m) -> [G6]
  Generator7/1(m) -> [G7]
  ES3/1(m) -> [G8]
  Generator9/1(m) -> [G9]
  Generator10/1(m) -> [G10]
  [G1] -> Bus Selector/1
  [G2] -> Bus Selector1/1
  [G3] -> Bus Selector2/1
  [G4] -> Bus Selector3/1
  [G6] -> Bus Selector5/1
  [G7] -> Bus Selector6/1
  [G8] -> Bus Selector7/1
  [G9] -> Bus Selector8/1
  [G10] -> Bus Selector9/1
  Bus Selector/1 -> Scope/1  "<f>"
  Bus Selector1/1 -> Scope/2  "<w>"
  Bus Selector2/1 -> Scope/3  "<f>"
  Bus Selector3/1 -> Scope/4  "<f>"
  Bus Selector5/1 -> Scope/5  "<w>"
  Bus Selector6/1 -> Scope/6  "<f>"
  Bus Selector7/1 -> Scope/7  "<w>"
  Bus Selector8/1 -> Scope/8  "<f>"
  Bus Selector9/1 -> Scope/9  "<f>"
  From10/1 -> Bus Selector10/1
  From11/1 -> Bus Selector11/1
  From12/1 -> Bus Selector12/1
  From13/1 -> Bus Selector13/1
  From14/1 -> Bus Selector14/1
  From15/1 -> Bus Selector15/1
  From16/1 -> Bus Selector16/1
  From17/1 -> Bus Selector17/1
  From18/1 -> Bus Selector18/1
  From19/1 -> Bus Selector19/1
  Bus Selector19/1 -> Scope1/10  "<delta>"
  Bus Selector18/1 -> Scope1/9  "<delta>"
  Bus Selector17/1 -> Scope1/8  "<delta>"
  Bus Selector16/1 -> Scope1/7  "<delta>"
  Bus Selector15/1 -> Scope1/6  "<delta>"
  Bus Selector14/1 -> Scope1/5  "<delta>"
  Bus Selector13/1 -> Scope1/4  "<delta>"
  Bus Selector12/1 -> Scope1/3  "<delta>"
  Bus Selector11/1 -> Scope1/2  "<delta>"
  Bus Selector10/1 -> Scope1/1  "<delta>"
  [G8] -> Bus Selector27/1
  [G1] -> Bus Selector20/1
  [G2] -> Bus Selector21/1
  [G7] -> Bus Selector26/1
  [G10] -> Bus Selector29/1
  [G9] -> Bus Selector28/1
  [G4] -> Bus Selector23/1
  [G3] -> Bus Selector22/1
  [G6] -> Bus Selector25/1
  [G5] -> Bus Selector24/1
  Bus Selector20/1 -> Scope2/1  "<Pe>"
  Bus Selector21/1 -> Scope2/2  "<Pe>"
  Bus Selector22/1 -> Scope2/3  "<Pe>"
  Bus Selector23/1 -> Scope2/4  "<Pe>"
  Bus Selector24/1 -> Scope2/5  "<Pwind>"
  Bus Selector25/1 -> Scope2/6  "<Pe>"
  Bus Selector26/1 -> Scope2/7  "<Pe>"
  Bus Selector27/1 -> Scope2/8  "<Pe>"
  Bus Selector28/1 -> Scope2/9  "<Pe>"
  Bus Selector29/1 -> Scope2/10  "<Pe>"
  Demux2/1 -> ES2/1(us_xy)
  Demux2/3 -> ES3/1(us_xy)
  Wind Generator - DFIG2/2(Igxy1) -> Mux14/1
  Wind Generator - DFIG2/3(GBxy) -> Mux14/2
  Wind Generator - DFIG1/3(GBxy) -> Mux15/2
  Wind Generator - DFIG1/2(Igxy1) -> Mux15/1
  Demux1/1 -> Wind Generator - DFIG1/2(Vsxy)
  Demux1/2 -> Wind Generator - DFIG2/2(Vsxy)
  Demux1/3 -> Generator1/1(Vgxy)
  Demux1/4 -> ES1/1(us_xy)
  Demux1/5 -> Generator3/1(Vgxy)
  Demux1/6 -> Generator4/1(Vgxy)
  Mux6/1 -> Mux3/7
  Mux5/1 -> Mux3/6
  Mux2/1 -> Mux3/5
  Mux1/1 -> Mux3/4
  Mux4/1 -> Mux3/3
  Mux14/1 -> Mux3/2
  Mux15/1 -> Mux3/1
  Constant/1 -> Wind Generator - DFIG2/1(Wind speed)
  Constant1/1 -> Wind Generator - DFIG1/1(Wind speed)
  Wind Generator - DFIG1/1(m) -> [G11]
  Wind Generator - DFIG2/1(m) -> [G12]
  Bus Selector30/1 -> Scope3/1  "<fw>"
  Bus Selector31/1 -> Scope3/2  "<fw>"
  [G11] -> Bus Selector30/1
  [G12] -> Bus Selector31/1
  Demux1/7 -> Wind Generator - DFIG3/2(Vsxy)
  Constant2/1 -> Wind Generator - DFIG3/1(Wind speed)
  Bus Selector4/1 -> ?  "<fw>"
  [G5] -> Bus Selector4/1

== system M10B39_es_V3/Network1 ==
  Ixy : Inport
  Clock : Clock
  Mux : Mux  Inputs=2
  S-Function : S-Function  FunctionName=TS_net_1_new  Parameters=YY_load,ng  SFunctionDeploymentMode=off  EnableBusSupport=off
  S-Function Examples : simulink/User-Defined Functions/S-Function Examples  Commented=on
  S-Function1 : S-Function  Commented=on  Parameters=YY_load,ng  SFunctionDeploymentMode=off  EnableBusSupport=off
  Vxy : Outport
  wires:
  Clock/1 -> Mux/1
  Ixy/1 -> Mux/2
  Mux/1 -> S-Function/1
  S-Function/1 -> Vxy/1
